simulink model "sampleModel1569_3_sub"  (R2023a)
settings: Solver=VariableStepAuto  StartTime=0.0  StopTime=10.0  RelTol=1e-3
libraries: hdlsllib x5, simulink x1
settings Model: Creator=user1  LastModifiedBy=user1
settings OptimizationCC: BlockReduction=off  ConditionallyExecuteInputs=off

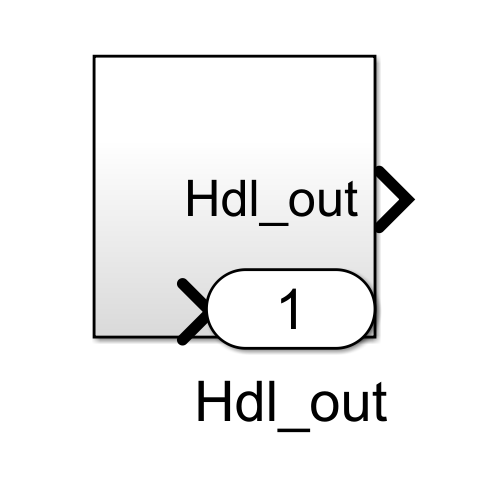
[thumbnail: Simulink's stored preview of the top-level diagram]
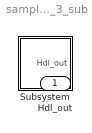
== system sampleModel1569_3_sub ==
  Subsystem : Subsystem
  Hdl_out : Outport  OutDataTypeStr=uint8

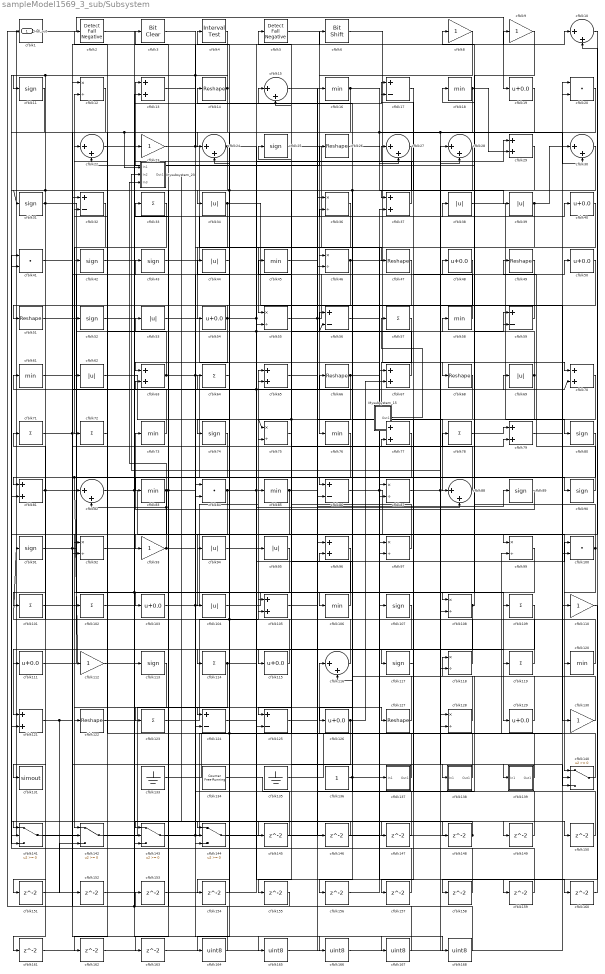
== system sampleModel1569_3_sub/Subsystem ==
  Mysubsystem_15 : Subsystem  TreatAsAtomicUnit=on  RTWFcnName=Mysubsystem_15
      settings: RTWFcnNameOpts=User specified  RTWFileNameOpts=Use function name
  Mysubsystem_23 : Subsystem  TreatAsAtomicUnit=on  RTWFcnName=Mysubsystem_23
      settings: RTWFcnNameOpts=User specified  RTWFileNameOpts=Use function name
  cfblk1 : ArithShift  BitShiftNumber=8
  cfblk{10,15,22,24,27..28,30,82,88,116} (10 alike) : Sum  Inputs=|++  OutDataTypeStr=uint8
  cfblk{20,41,84,100} (4 alike) : DotProduct  OutDataTypeStr=uint8
  cfblk{33,57,64,71..72,78,101..102,109,114,119,123} (12 alike) : Sum  Inputs=+  OutDataTypeStr=uint8
  cfblk{19,40,48,50,54,103,111,115,126,129} (10 alike) : Bias  Bias=0.0  SaturateOnIntegerOverflow=off
  cfblk{34,38..39,44,53,62,69,94..95,104} (10 alike) : Abs  OutDataTypeStr=uint8  SaturateOnIntegerOverflow=off
  cfblk{13,29,37,63,65,67,70,77,79,81,96,105,121} (13 alike) : Sum  OutDataTypeStr=uint8
  cfblk{16,18,45,58,61,73,76,83,85,106,120} (11 alike) : MinMax  OutDataTypeStr=uint8
  cfblk{11,25,31,42..43,52,74,80,89..91,107,113,117} (14 alike) : Signum
  cfblk{12,36,46,55,75,87,92,97,99,108,118,128} (12 alike) : Product  Inputs=*/  OutDataTypeStr=uint8  RndMeth=Zero  SaturateOnIntegerOverflow=on
  cfblk{8..9,23,93,110,112,130} (7 alike) : Gain  OutDataTypeStr=uint8
  cfblk{14,26,47,49,51,66,68,122,127} (9 alike) : Reshape
  cfblk{17,32,56,59,86,124..125} (7 alike) : Sum  Inputs=+-  OutDataTypeStr=uint8
  cfblk131 : ToWorkspace  VariableName=simout  SaveFormat=Timeseries  SampleTime=-1
  cfblk133 : Ground
  cfblk134 : hdlsllib/Sources/Counter Free-Running  NumBits=16  tsamp=-1
  cfblk135 : Ground
  cfblk136 : Constant  OutDataTypeStr=uint8  SampleTime=-1
  cfblk137 : Subsystem
      settings: LibrarySourceBlock=|
      | hdlsllib/Ports &
      | Subsystems/Subsystem
  cfblk138 : Subsystem
      settings: LibrarySourceBlock=|
      | hdlsllib/Ports &
      | Subsystems/Subsystem
  cfblk139 : Subsystem
      settings: LibrarySourceBlock=|
      | hdlsllib/Ports &
      | Subsystems/Subsystem
  cfblk{140..144} (5 alike) : Switch  OutDataTypeStr=uint8  SaturateOnIntegerOverflow=off  InputSameDT=off
  cfblk{145..163} (19 alike) : Delay  SampleTime=1
  cfblk{164..168} (5 alike) : DataTypeConversion  OutDataTypeStr=uint8  SaturateOnIntegerOverflow=off  RndMeth=Floor
  cfblk2 : hdlsllib/Logic and Bit Operations/Detect Fall Negative  vinit=0  OutDataTypeStr=uint8
  cfblk3 : simulink/Logic and Bit Operations/Bit Clear  iBit=0
      settings: LibrarySourceBlock=|
      | hdlsllib/Logic and Bit
      | Operations/Bit Clear
  cfblk4 : hdlsllib/Logic and Bit Operations/Interval Test  IntervalClosedRight=on  uplimit=0.5  IntervalClosedLeft=on  lowlimit=-0.5  OutDataTypeStr=uint8
  cfblk5 : hdlsllib/Logic and Bit Operations/Detect Fall Negative  vinit=0  OutDataTypeStr=uint8
  cfblk6 : hdlsllib/Logic and Bit Operations/Bit Shift  mode=Shift Left Logical  N=0
  Hdl_out : Outport  OutDataTypeStr=uint8
  wires:
  cfblk91/1 -> cfblk9/1, cfblk48/1
  cfblk87/1 -> cfblk140/3, Mysubsystem_23/2(In2)
  cfblk5/1 -> cfblk76/1
  cfblk29/1 -> cfblk145/1, cfblk75/1
  cfblk118/1 -> cfblk44/1, cfblk91/1
  cfblk107/1 -> cfblk117/1
  cfblk37/1 -> cfblk13/1
  cfblk138/1(Out1) -> cfblk116/1
  cfblk104/1 -> cfblk129/1
  cfblk46/1 -> cfblk123/1, cfblk70/1
  cfblk10/1 -> cfblk93/1
  cfblk134/1 -> cfblk118/1
  cfblk89/1 -> cfblk73/1
  cfblk54/1 -> cfblk143/3, cfblk51/1, cfblk6/1, cfblk160/1, cfblk56/2
  cfblk99/1 -> cfblk106/1
  cfblk119/1 -> cfblk65/1
  cfblk121/1 -> cfblk152/1, cfblk75/2
  cfblk108/1 -> cfblk125/2, cfblk8/1
  cfblk63/1 -> cfblk2/1, cfblk127/1, cfblk137/1(In1)
  cfblk84/1 -> cfblk142/1, cfblk77/2, cfblk119/1
  cfblk22/1 -> cfblk113/1
  cfblk8/1 -> cfblk46/1
  cfblk127/1 -> cfblk14/1
  cfblk36/1 -> cfblk55/1
  cfblk141/1 -> cfblk43/1
  cfblk68/1 -> cfblk86/1
  cfblk136/1 -> cfblk58/1, cfblk66/1
  cfblk39/1 -> cfblk114/1, cfblk30/1
  cfblk66/1 -> cfblk59/1, cfblk86/2
  cfblk111/1 -> cfblk64/1
  cfblk50/1 -> cfblk118/2
  cfblk82/1 -> cfblk56/1, cfblk140/1
  cfblk100/1 -> cfblk22/2, cfblk120/1
  cfblk47/1 -> cfblk115/1
  cfblk125/1 -> cfblk46/2
  cfblk123/1 -> cfblk105/1
  cfblk6/1 -> cfblk68/1
  cfblk124/1 -> cfblk95/1
  cfblk103/1 -> cfblk78/1, cfblk85/1
  cfblk93/1 -> cfblk59/2, cfblk82/2, Mysubsystem_23/3(In3)
  cfblk38/1 -> cfblk80/1
  cfblk97/1 -> cfblk15/1
  cfblk51/1 -> cfblk109/1
  cfblk78/1 -> cfblk79/1
  cfblk23/1 -> cfblk10/1, cfblk47/1
  cfblk96/1 -> cfblk103/1
  cfblk94/1 -> cfblk70/2, cfblk29/1
  cfblk102/1 -> cfblk17/1
  cfblk19/1 -> cfblk24/1
  cfblk57/1 -> cfblk77/1
  cfblk31/1 -> cfblk131/1, cfblk90/1
  cfblk83/1 -> cfblk121/2, cfblk33/1, cfblk50/1
  cfblk58/1 -> cfblk27/1
  cfblk88/1 -> cfblk25/1
  cfblk25/1 -> cfblk97/1
  cfblk112/1 -> cfblk40/1
  cfblk142/1 -> cfblk124/1
  cfblk101/1 -> cfblk53/1
  cfblk143/1 -> cfblk79/2, cfblk110/1
  cfblk133/1 -> cfblk67/1
  cfblk1/1 -> cfblk19/1
  cfblk2/1 -> cfblk165/1, cfblk108/2
  cfblk4/1 -> cfblk124/2, cfblk141/3, cfblk141/1
  cfblk109/1 -> cfblk121/1
  cfblk67/1 -> cfblk5/1
  cfblk137/1(Out1) -> cfblk32/2, cfblk4/1
  cfblk81/1 -> cfblk161/1, cfblk112/1
  cfblk73/1 -> cfblk12/2
  cfblk14/1 -> cfblk92/2, cfblk11/1
  cfblk33/1 -> cfblk72/1
  cfblk32/1 -> cfblk42/1
  cfblk30/1 -> cfblk126/1, cfblk111/1
  cfblk52/1 -> cfblk26/1
  cfblk13/1 -> cfblk138/1(In1)
  cfblk86/1 -> cfblk159/1, cfblk99/1
  cfblk34/1 -> cfblk144/3, cfblk130/1
  cfblk28/1 -> cfblk34/1
  cfblk56/1 -> cfblk140/2
  cfblk71/1 -> cfblk139/1(In1), cfblk69/1
  cfblk113/1 -> cfblk122/1
  cfblk26/1 -> cfblk27/2
  cfblk48/1 -> cfblk81/1
  cfblk120/1 -> cfblk105/2
  cfblk53/1 -> cfblk107/1
  cfblk11/1 -> cfblk81/2
  cfblk80/1 -> cfblk125/1
  cfblk126/1 -> cfblk155/1, cfblk67/2
  cfblk135/1 -> cfblk99/2
  cfblk42/1 -> cfblk84/2
  cfblk106/1 -> cfblk65/2
  cfblk139/1(Out1) -> cfblk15/2
  cfblk74/1 -> cfblk151/1, cfblk82/1
  cfblk75/1 -> cfblk45/1
  cfblk128/1 -> cfblk23/1
  cfblk44/1 -> cfblk144/1
  cfblk62/1 -> cfblk88/1
  cfblk41/1 -> cfblk83/1
  cfblk129/1 -> cfblk61/1
  cfblk76/1 -> cfblk144/2
  cfblk114/1 -> cfblk143/1, cfblk100/1
  cfblk85/1 -> cfblk38/1, cfblk104/1
  cfblk144/1 -> cfblk87/1
  cfblk17/1 -> cfblk37/1
  cfblk105/1 -> cfblk89/1
  cfblk130/1 -> cfblk96/2
  cfblk79/1 -> cfblk100/2
  cfblk18/1 -> cfblk29/2, cfblk128/2, cfblk94/1
  cfblk24/1 -> cfblk88/2, cfblk63/1
  cfblk95/1 -> cfblk102/1
  cfblk16/1 -> cfblk39/1, cfblk30/2, cfblk92/1, Mysubsystem_23/1(In1)
  cfblk59/1 -> cfblk52/1
  cfblk115/1 -> cfblk62/1
  cfblk69/1 -> cfblk97/2, cfblk18/1
  cfblk65/1 -> cfblk16/1
  cfblk140/1 -> cfblk22/1
  cfblk40/1 -> cfblk54/1
  cfblk116/1 -> cfblk71/1
  cfblk90/1 -> cfblk49/1
  cfblk9/1 -> cfblk108/1
  cfblk55/1 -> cfblk87/2, cfblk28/2
  cfblk12/1 -> cfblk101/1, cfblk31/1
  cfblk3/1 -> cfblk168/1
  cfblk27/1 -> cfblk41/2, cfblk74/1
  cfblk43/1 -> cfblk36/2
  cfblk145/1 -> cfblk84/1
  cfblk45/1 -> cfblk146/1
  cfblk146/1 -> cfblk141/2
  cfblk70/1 -> cfblk147/1
  cfblk147/1 -> cfblk116/2
  cfblk15/1 -> cfblk148/1
  cfblk148/1 -> Hdl_out/1, cfblk142/2
  cfblk149/1 -> cfblk96/1
  cfblk122/1 -> cfblk150/1
  cfblk150/1 -> cfblk17/2
  cfblk151/1 -> cfblk142/3
  cfblk152/1 -> cfblk13/2
  cfblk153/1 -> cfblk55/2
  cfblk64/1 -> cfblk154/1
  cfblk154/1 -> cfblk24/2
  cfblk155/1 -> cfblk1/1
  cfblk49/1 -> cfblk156/1
  cfblk156/1 -> cfblk37/2
  cfblk117/1 -> cfblk157/1
  cfblk157/1 -> cfblk12/1
  cfblk110/1 -> cfblk158/1
  cfblk158/1 -> cfblk41/1
  cfblk159/1 -> cfblk63/2
  cfblk160/1 -> cfblk10/2
  cfblk161/1 -> cfblk128/1
  cfblk72/1 -> cfblk162/1
  cfblk162/1 -> cfblk36/1
  cfblk77/1 -> cfblk163/1
  cfblk163/1 -> cfblk28/1
  cfblk20/1 -> cfblk164/1
  cfblk164/1 -> cfblk153/1
  cfblk165/1 -> cfblk20/1
  cfblk92/1 -> cfblk166/1
  cfblk166/1 -> cfblk20/2
  cfblk61/1 -> cfblk167/1
  cfblk167/1 -> cfblk3/1
  cfblk168/1 -> cfblk32/1, cfblk143/2
  Mysubsystem_15/1(Out1) -> cfblk57/1
  Mysubsystem_23/1(Out1) -> cfblk149/1

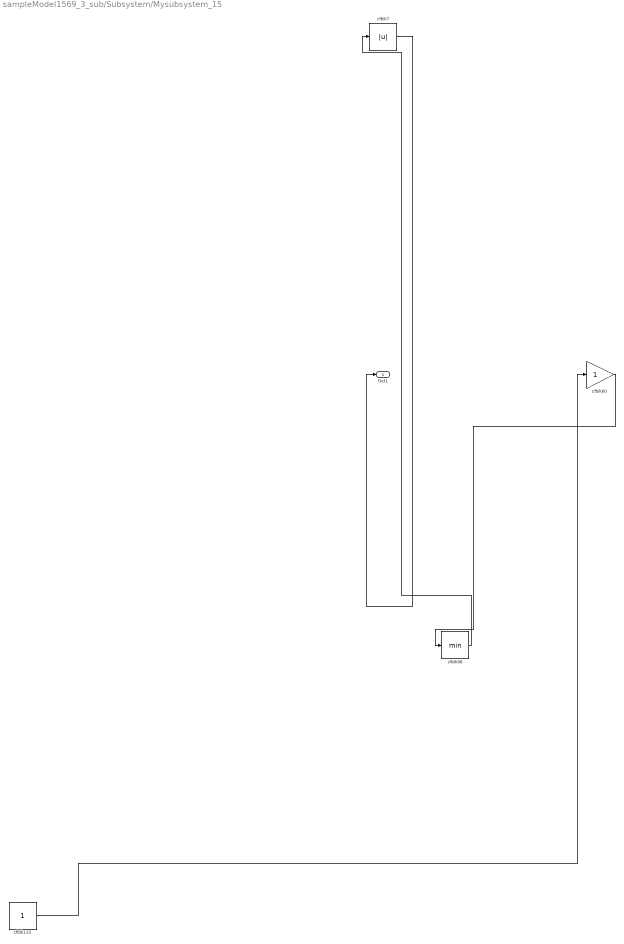
== system sampleModel1569_3_sub/Subsystem/Mysubsystem_15 ==
  cfblk132 : Constant  SampleTime=-1
  cfblk60 : Gain
  cfblk7 : Abs  SaturateOnIntegerOverflow=off
  cfblk98 : MinMax
  Out1 : Outport
  wires:
  cfblk7/1 -> Out1/1
  cfblk98/1 -> cfblk7/1
  cfblk60/1 -> cfblk98/1
  cfblk132/1 -> cfblk60/1

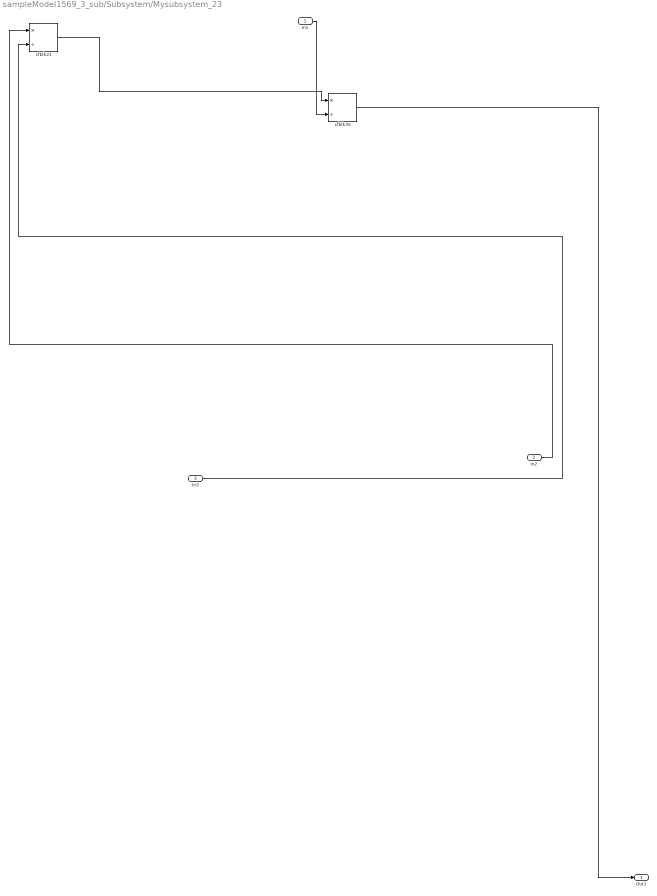
== system sampleModel1569_3_sub/Subsystem/Mysubsystem_23 ==
  In1 : Inport
  In2 : Inport  Port=2
  In3 : Inport  Port=3
  cfblk21 : Product  Inputs=*/  RndMeth=Zero  SaturateOnIntegerOverflow=on
  cfblk35 : Product  Inputs=*/  RndMeth=Zero  SaturateOnIntegerOverflow=on
  Out1 : Outport
  wires:
  cfblk35/1 -> Out1/1
  In3/1 -> cfblk21/2
  In2/1 -> cfblk21/1
  In1/1 -> cfblk35/2
  cfblk21/1 -> cfblk35/1

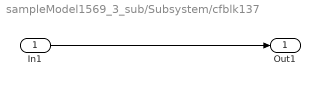
== system sampleModel1569_3_sub/Subsystem/cfblk137 ==
  In1 : Inport
  Out1 : Outport
  wires:
  In1/1 -> Out1/1

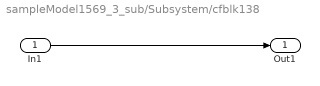
== system sampleModel1569_3_sub/Subsystem/cfblk138 ==
  In1 : Inport
  Out1 : Outport
  wires:
  In1/1 -> Out1/1

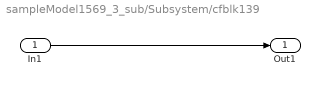
== system sampleModel1569_3_sub/Subsystem/cfblk139 ==
  In1 : Inport
  Out1 : Outport
  wires:
  In1/1 -> Out1/1
